simulink model "bcm"  (R2019b)
settings: Solver=FixedStepAuto  StartTime=0.0  StopTime=10.0  FixedStep=0.1  RelTol=1e-3
settings Model: Creator=ADEMATO1  LastModifiedBy=EMORAI12
settings SolverCC: PositivePriorityOrder=on  AutoInsertRateTranBlk=on  InsertRTBMode=Always

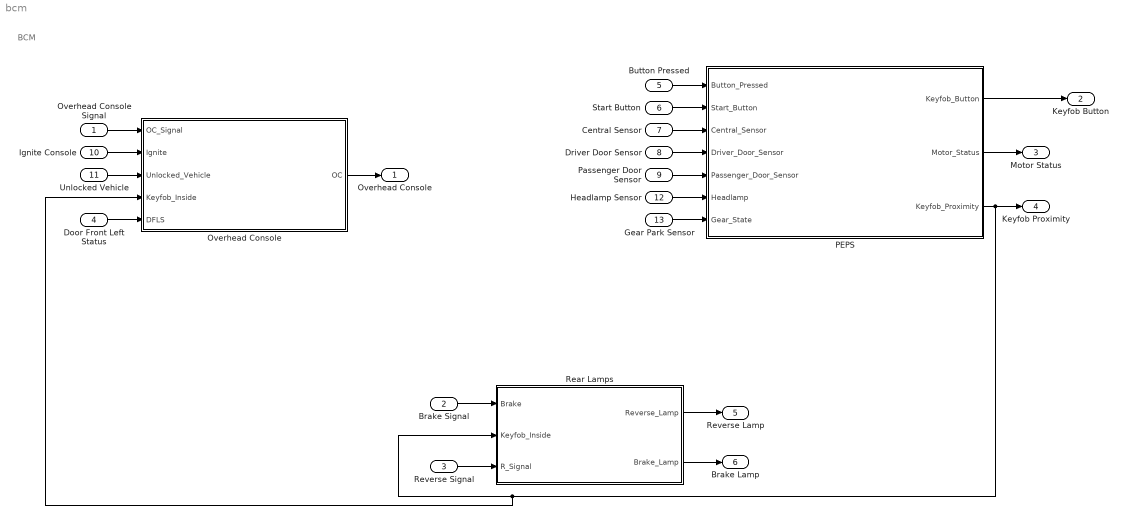
== system bcm ==
  note: BCM
  Overhead Console Signal : Inport
  Brake Signal : Inport  Port=2
  Reverse Signal : Inport  Port=3
  Door Front Left Status : Inport  Port=4
  Button Pressed : Inport  Port=5
  Start Button : Inport  Port=6
  Central Sensor : Inport  Port=7
  Driver Door Sensor : Inport  Port=8
  Passenger Door Sensor : Inport  Port=9
  Ignite Console : Inport  Port=10
  Unlocked Vehicle : Inport  Port=11
  Headlamp Sensor : Inport  Port=12
  Gear Park Sensor : Inport  Port=13
  Overhead Console : Stateflow chart  TreatAsAtomicUnit=on
  PEPS : Stateflow chart  TreatAsAtomicUnit=on
  Rear Lamps : Stateflow chart  TreatAsAtomicUnit=on
  "  Overhead Console  " : Outport
  Keyfob Button : Outport  Port=2
  Motor Status : Outport  Port=3
  Keyfob Proximity : Outport  Port=4
  Reverse Lamp : Outport  Port=5
  Brake Lamp : Outport  Port=6
  wires:
  Headlamp Sensor/1 -> PEPS/6(Headlamp)
  PEPS/2(Motor_Status) -> Motor Status/1
  Gear Park Sensor/1 -> PEPS/7(Gear_State)
  Brake Signal/1 -> Rear Lamps/1(Brake)
  Rear Lamps/2(Brake_Lamp) -> Brake Lamp/1
  Overhead Console Signal/1 -> Overhead Console/1(OC_Signal)
  Reverse Signal/1 -> Rear Lamps/3(R_Signal)
  Ignite Console/1 -> Overhead Console/2(Ignite)
  Door Front Left Status/1 -> Overhead Console/5(DFLS)
  Button Pressed/1 -> PEPS/1(Button_Pressed)
  Passenger Door Sensor/1 -> PEPS/5(Passenger_Door_Sensor)
  Driver Door Sensor/1 -> PEPS/4(Driver_Door_Sensor)
  Central Sensor/1 -> PEPS/3(Central_Sensor)
  Start Button/1 -> PEPS/2(Start_Button)
  Rear Lamps/1(Reverse_Lamp) -> Reverse Lamp/1
  Overhead Console/1(OC) -> "  Overhead Console  "/1
  Unlocked Vehicle/1 -> Overhead Console/3(Unlocked_Vehicle)
  PEPS/1(Keyfob_Button) -> Keyfob Button/1
  PEPS/3(Keyfob_Proximity) -> Overhead Console/4(Keyfob_Inside), Rear Lamps/2(Keyfob_Inside), Keyfob Proximity/1

== stateflow chart bcm/Overhead Console ==
  state state_ic
    during :
    OC = 1;
  state Initial_State
    entry:
    OC = 0;
  state OC_On_Initial
    during:
    OC = 1;
  state Overhead_Console
    during:
    if (OC_Signal == 1)
    OC = 1;
    elseif (OC_Signal == 0)
    OC = 0;
    end
  state OC_Off1
    entry:
    OC = 0;
  Overhead_Console -> Initial_State [order 2] : [Unlocked_Vehicle == 0]
  (default) -> Initial_State
  state_ic -> OC_Off1 [order 1] : after(10,sec)
  Overhead_Console -> state_ic [order 1] : [(hasChangedTo(Keyfob_Inside,0) == 1 & Ignite == 0 & DFLS == 0)]
  Initial_State -> OC_On_Initial : [Unlocked_Vehicle==1& DFLS == 0]
  OC_On_Initial -> Overhead_Console : after(2,sec)
  state_ic -> Overhead_Console [order 2] : [DFLS == 1]
  OC_Off1 -> OC_On_Initial [order 1] : [hasChangedTo(Unlocked_Vehicle,1) == 1 & DFLS == 0 ]
  OC_Off1 -> Overhead_Console [order 2] : [(DFLS == 1 || hasChangedTo(Keyfob_Inside,1) == 1)]
  data: OC_Signal input; Ignite input; Unlocked_Vehicle input; Keyfob_Inside input; OC output; DFLS input; r_Keyfob_Inside local; data local

== stateflow chart bcm/Rear Lamps ==
  state Rear_Lamps
    state Brake_Lamp_Enable [parallel]
      during:
      if (Keyfob_Inside == 1 & Brake == 1)
      Brake_Lamp = 1;
      else
      Brake_Lamp = 0;
      end
      settings: executionOrder=1
    state Reverse_Enable [parallel]
      during:
      if (R_Signal == 4)
      Reverse_Lamp = 1;
      else
      Reverse_Lamp = 0;
      end
      settings: executionOrder=2
  data: Brake input; Keyfob_Inside input; R_Signal input; Reverse_Lamp output; Brake_Lamp output

== stateflow chart bcm/PEPS ==
  state PEPS
    state PEPS_Smart_Key [parallel]
      entry:
      Motor_Status = 0;
      during:
      Ignite = Start_Button;
      if (Ignite == 1 & Keyfob_Proximity == 1 & Gear_State == 1)
      Motor_Status = 1;
      elseif (Ignite == 0 & Headlamp == 0 & Gear_State == 1)
      Motor_Status = 0;
      end
      settings: executionOrder=3
    state PEPS_Keyfob [parallel]
      entry:
      Keyfob_Button = 0;
      during:
      Keyfob_Button = Button_Pressed;
      if (Button_Pressed == 1)
      Keyfob_Button = 1;
      elseif (Button_Pressed == 2)
      Keyfob_Button = 2;
      end
      settings: executionOrder=2
    state PEPS_Sattelite [parallel]
      during:
      S1 = Driver_Door_Sensor;
      S2 = Central_Sensor;
      S3 = Passenger_Door_Sensor;
      if (S1 <= 2 & S3 <= 2 & S2 <= 1.5)
      Keyfob_Proximity = 1;
      else
      Keyfob_Proximity = 0;
      end
      settings: executionOrder=1
  data: Button_Pressed input; Keyfob_Button output; Start_Button input; Central_Sensor input; Driver_Door_Sensor input; Passenger_Door_Sensor input; Motor_Status output; Keyfob_Proximity output; S3 local; S1 local; S2 local; Headlamp input; Gear_State input; Ignite local
